simulink model "ejercicio"  (R2015a)
settings: Solver=ode45  StartTime=0.0  StopTime=.1  RelTol=1e-3
values from neighbouring files (symbols this model uses):
  B = [0;1/m]    [ejercicio.m]
  R = 1e5    (= 100000)    [practica1t.m]    (also in practica2t.m)
undefined symbols (not defined in the file or in its folder): J, K, L
settings Model: Creator=Sala2  LastModifiedBy=Sala2

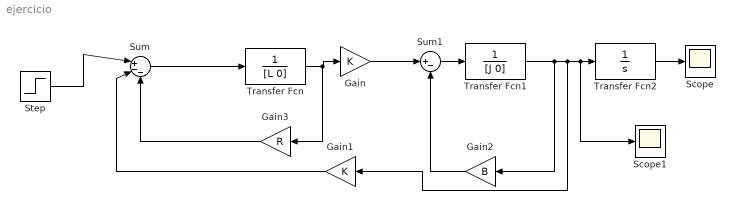
== system ejercicio ==
  Gain : Gain  Gain=K
  Gain1 : Gain  Gain=K
  Gain2 : Gain  Gain=B
  Gain3 : Gain  Gain=R
  Scope : Scope
      settings: YMin=0  YMax=100
  Scope1 : Scope
      settings: YMin=35.819  YMax=35.83
  Step : Step  Time=0  SampleTime=0
  Sum : Sum  Inputs=|+--
  Sum1 : Sum  Inputs=|+-
  Transfer Fcn : TransferFcn  Denominator=[L 0]
  Transfer Fcn1 : TransferFcn  Denominator=[J 0]
  Transfer Fcn2 : TransferFcn  Denominator=[1 0]
  wires:
  Sum/1 -> Transfer Fcn/1
  Gain/1 -> Sum1/1
  Transfer Fcn/1 -> Gain3/1, Gain/1
  Sum1/1 -> Transfer Fcn1/1
  Transfer Fcn2/1 -> Scope/1
  Gain2/1 -> Sum1/2
  Transfer Fcn1/1 -> Gain1/1, Scope1/1, Transfer Fcn2/1, Gain2/1
  Gain1/1 -> Sum/2
  Gain3/1 -> Sum/3
  Step/1 -> Sum/1
